simulink subsystem "Motors"  (R2024a)
settings: Solver=VariableStepAuto  StartTime=0.0  StopTime=10.0  RelTol=1e-3
libraries: stm32l4xxblockslib x2, stm32f4xxblockslib x1
settings Model: Creator=JesseJabezArendse  LastModifiedBy=griff
settings RTWCC: GPUComputeCapability=3.5

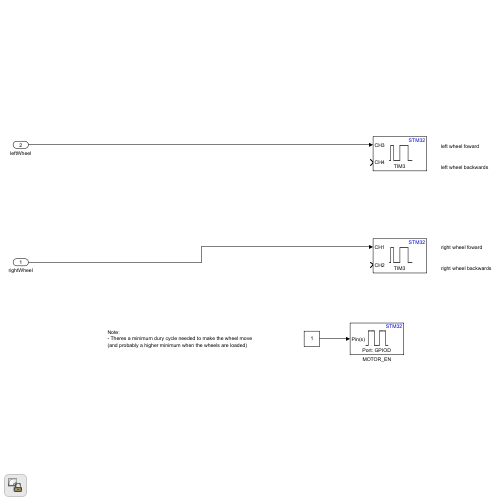
[thumbnail: Simulink's stored preview of the top-level diagram]
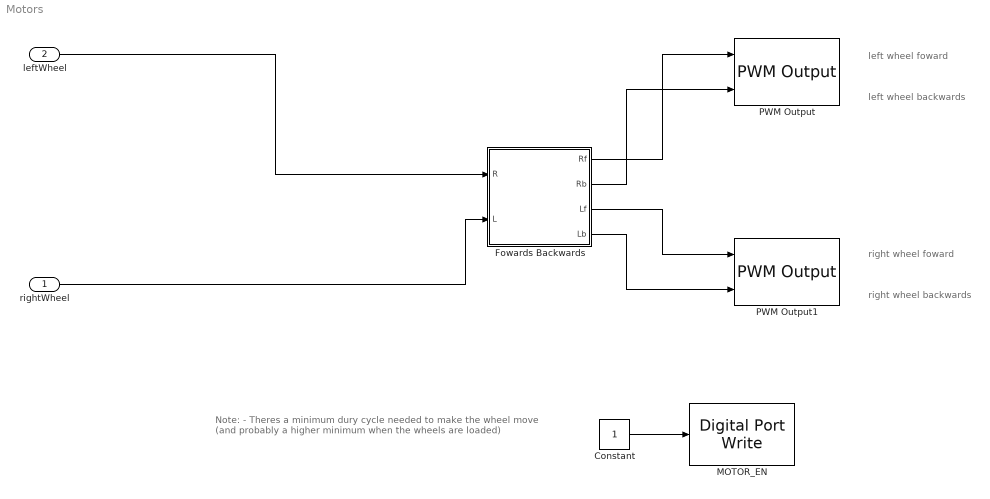
== system Motors ==
  note: Note:
      | - Theres a minimum dury cycle needed to make the wheel move (and probably a higher minimum when the wheels are loaded)
  note: left wheel foward
  note: left wheel backwards
  note: right wheel backwards
  note: right wheel foward
  rightWheel : Inport
  leftWheel : Inport  Port=2
  Constant : Constant
  Fowards Backwards : MATLAB Function  TreatAsAtomicUnit=on
  MOTOR_EN : stm32f4xxblockslib/Digital Port Write  PortName=GPIOD  PinNumber=7  ReadOperation=off  IOAsArray=on  EnableSimPort=off  hoistedMaskSrc=ECSoC/ECSimCodegen/Digital Port Write
      settings: LibrarySourceBlock=stm32l4xxblockslib/Digital Port Write
  PWM Output : stm32l4xxblockslib/PWM Output  TimerModule=TIM3  DutycycleUnits=Percentage  EnableChannel1=off  EnableChannel2=off  EnableChannel3=on  EnableChannel4=on  EnableChannel5=off  EnableChannel6=off  EnableCounterInput=off  EnableMainOutputInput=off  EnableFrequencyInput=off  SetRCAfterCE=off  OutputDirection=off  OutputMainOutputEnableStatus=off  SampleTime=0.1  EnableSimPort=off  EnableUpdateEvent=off  EnableCaptureCompare1Event=off  EnableCaptureCompare2Event=off  EnableCaptureCompare3Event=off  EnableCaptureCompare4Event=off  EnableTriggerEvent=off  EnableBreakEvent=off  EnableBreakEvent2=off  ProcessorFamily=STM32L4  hoistedMaskSrc=ECSoC/ECSimCodegen/PWM Output
  PWM Output1 : stm32l4xxblockslib/PWM Output  TimerModule=TIM3  DutycycleUnits=Percentage  EnableChannel1=on  EnableChannel2=on  EnableChannel3=off  EnableChannel4=off  EnableChannel5=off  EnableChannel6=off  EnableCounterInput=off  EnableMainOutputInput=off  EnableFrequencyInput=off  SetRCAfterCE=off  OutputDirection=off  OutputMainOutputEnableStatus=off  SampleTime=0.1  EnableSimPort=off  EnableUpdateEvent=off  EnableCaptureCompare1Event=off  EnableCaptureCompare2Event=off  EnableCaptureCompare3Event=off  EnableCaptureCompare4Event=off  EnableTriggerEvent=off  EnableBreakEvent=off  EnableBreakEvent2=off  ProcessorFamily=STM32L4  hoistedMaskSrc=ECSoC/ECSimCodegen/PWM Output
  wires:
  Constant/1 -> MOTOR_EN/1
  leftWheel/1 -> Fowards Backwards/1(R)
  rightWheel/1 -> Fowards Backwards/2(L)
  Fowards Backwards/1(Rf) -> PWM Output/1
  Fowards Backwards/2(Rb) -> PWM Output/2
  Fowards Backwards/3(Lf) -> PWM Output1/1
  Fowards Backwards/4(Lb) -> PWM Output1/2

== matlab function Motors/Fowards Backwards ==
  data: R input; Rf output; L input; Rb output; Lf output; Lb output
function [Rf,Rb,Lf,Lb] = fcn(R,L)
persistent Rmem
persistent Lmem

if isempty(Rmem)
    Rmem=R;
end
if isempty(Lmem)
    Lmem=L;
end





Rmem=0.2*Rmem+0.8*R;
Lmem=0.2*Lmem+0.8*L;


if Rmem>10
    Rf=Rmem/3+66;
    Rb=0;

elseif Rmem<-10
    Rf=0;
    Rb=abs(Rmem/3-66);
else 
    Rf=0;
    Rb=0;
end


if Lmem>10
    Lf=Lmem/3+66;
    Lb=0;

elseif Lmem<-10
    Lf=0;
    Lb=abs(Lmem/3-66);
else 
    Lf=0;
    Lb=0;
end

end
